simulink model "Hw6P1b1"  (R2017b)
settings: Solver=FixedStepAuto  StartTime=0.0  StopTime=10.0  FixedStep=0.01  RelTol=1e-3
undefined symbols (not defined in the file or in its folder): omega, zeta
libraries: fuzblock x4
settings Model: Creator=Soutrik  LastModifiedBy=Gopanraj
settings CodeAppCC: StateflowObjectComments=on

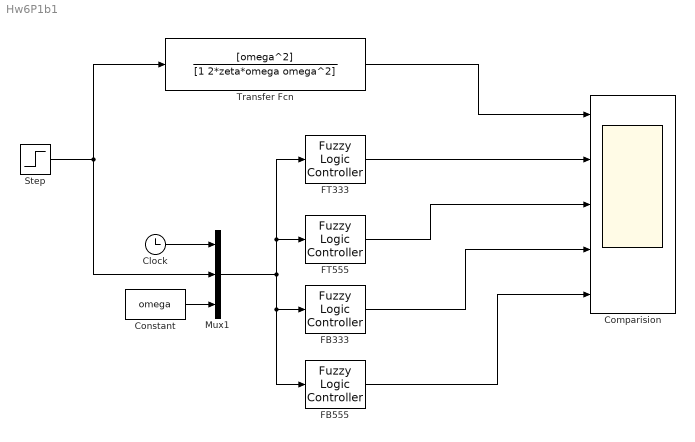
== system Hw6P1b1 ==
  Clock : Clock
  Comparision : Scope  NumInputPorts=5
  Constant : Constant  Value=omega
  FB333 : fuzblock/Fuzzy Logic  Controller  FIS=fb333  OutputSampleNumber=101  DataType=double  FuzzifiedInputs=off  RuleFiringStrengths=off  RuleOutputs=off  AggregatedOutputs=off  SimulateUsing=Interpreted execution
  FB555 : fuzblock/Fuzzy Logic  Controller  FIS=fb555  OutputSampleNumber=101  DataType=double  FuzzifiedInputs=off  RuleFiringStrengths=off  RuleOutputs=off  AggregatedOutputs=off  SimulateUsing=Interpreted execution
  FT333 : fuzblock/Fuzzy Logic  Controller  FIS=ft333  OutputSampleNumber=101  DataType=double  FuzzifiedInputs=off  RuleFiringStrengths=off  RuleOutputs=off  AggregatedOutputs=off  SimulateUsing=Interpreted execution
  FT555 : fuzblock/Fuzzy Logic  Controller  FIS=ft555  OutputSampleNumber=101  DataType=double  FuzzifiedInputs=off  RuleFiringStrengths=off  RuleOutputs=off  AggregatedOutputs=off  SimulateUsing=Interpreted execution
  Mux1 : Mux  Inputs=3
  Step : Step  SampleTime=0
  Transfer Fcn : TransferFcn  Numerator=[omega^2]  Denominator=[1 2*zeta*omega omega^2]
  wires:
  Step/1 -> Mux1/2, Transfer Fcn/1
  Clock/1 -> Mux1/1
  Constant/1 -> Mux1/3
  Mux1/1 -> FT333/1, FT555/1, FB333/1, FB555/1
  Transfer Fcn/1 -> Comparision/1
  FT333/1 -> Comparision/2
  FT555/1 -> Comparision/3
  FB333/1 -> Comparision/4
  FB555/1 -> Comparision/5
